simulink model "ans17"  (R2019a)
settings: Solver=VariableStepAuto  StartTime=0.0  StopTime=10.0  RelTol=1e-3
undefined symbols (not defined in the file or in its folder): a4, d1, feff, J_eff, KD, KI, KP, kT, n, TL
settings Model: Creator=andylei  LastModifiedBy=matth
settings DataIOCC: SaveFormat=StructureWithTime  ReturnWorkspaceOutputs=off
settings DebuggingCC: ArithmeticOperatorsInVariantConditions=warning

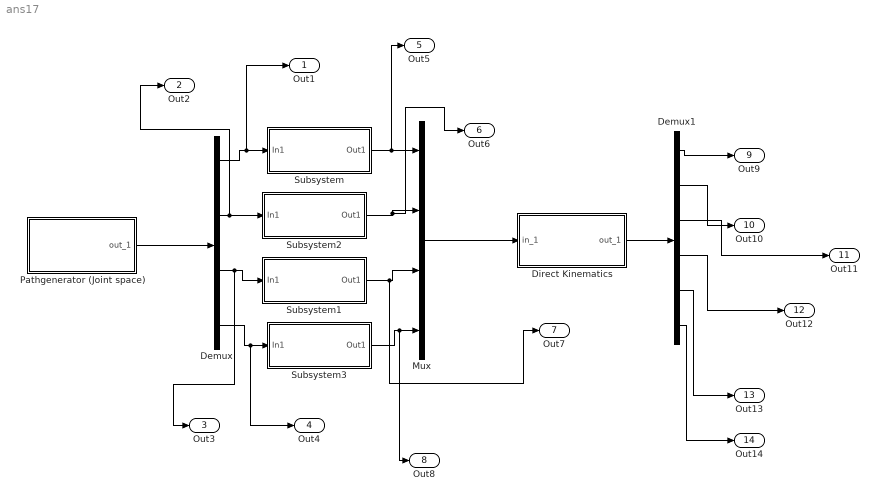
== system ans17 ==
  Demux : Demux
  Demux1 : Demux  Outputs=6
  Direct Kinematics : Subsystem
      mask Display: disp('Alto-Robot')
  Mux : Mux
  Pathgenerator (Joint space) : Subsystem
      mask Display: disp('Alto-Robot\n path -> q')
  Subsystem : Subsystem
  Subsystem1 : Subsystem
  Subsystem2 : Subsystem
  Subsystem3 : Subsystem
  Out1 : Outport
  Out2 : Outport  Port=2
  Out3 : Outport  Port=3
  Out4 : Outport  Port=4
  Out5 : Outport  Port=5
  Out6 : Outport  Port=6
  Out7 : Outport  Port=7
  Out8 : Outport  Port=8
  Out9 : Outport  Port=9
  Out10 : Outport  Port=10
  Out11 : Outport  Port=11
  Out12 : Outport  Port=12
  Out13 : Outport  Port=13
  Out14 : Outport  Port=14
  wires:
  Pathgenerator (Joint space)/1(out_1) -> Demux/1
  Mux/1 -> Direct Kinematics/1(in_1)
  Demux/1 -> Out1/1, Subsystem/1(In1)
  Demux/2 -> Subsystem2/1(In1), Out2/1
  Demux/3 -> Out3/1, Subsystem1/1(In1)
  Demux/4 -> Out4/1, Subsystem3/1(In1)
  Subsystem/1(Out1) -> Out5/1, Mux/1
  Subsystem2/1(Out1) -> Out6/1, Mux/2
  Subsystem1/1(Out1) -> Out7/1, Mux/3
  Subsystem3/1(Out1) -> Out8/1, Mux/4
  Direct Kinematics/1(out_1) -> Demux1/1
  Demux1/1 -> Out9/1
  Demux1/2 -> Out10/1
  Demux1/3 -> Out11/1
  Demux1/4 -> Out12/1
  Demux1/5 -> Out13/1
  Demux1/6 -> Out14/1

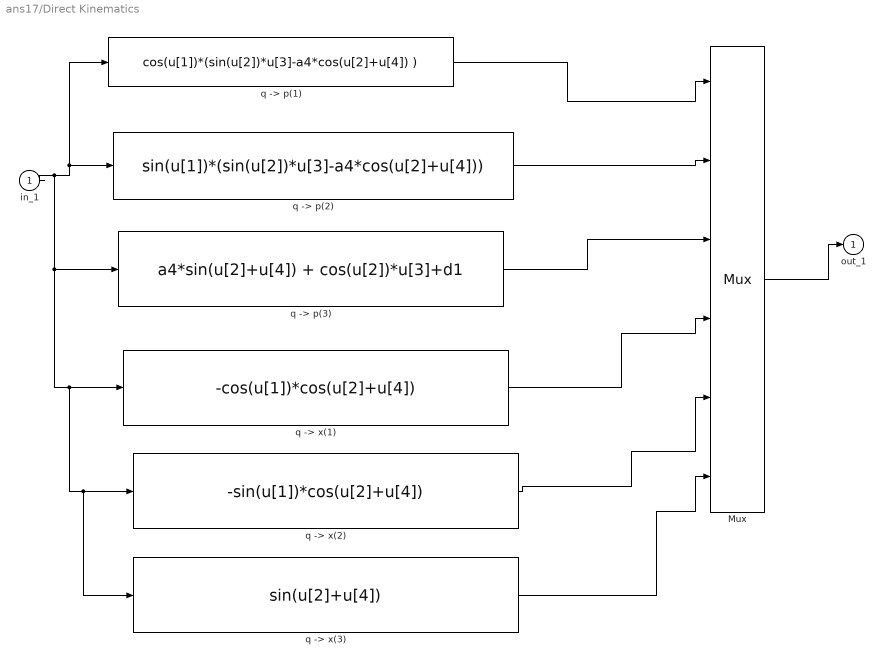
== system ans17/Direct Kinematics ==
  in_1 : Inport
  Mux : Mux  Inputs=6
  "q -> p(1)" : Fcn  Expr=cos(u[1])*(sin(u[2])*u[3]-a4*cos(u[2]+u[4]) )
  "q -> p(2)" : Fcn  Expr=sin(u[1])*(sin(u[2])*u[3]-a4*cos(u[2]+u[4]))
  "q -> p(3)" : Fcn  Expr=a4*sin(u[2]+u[4]) + cos(u[2])*u[3]+d1
  "q -> x(1)" : Fcn  Expr=-cos(u[1])*cos(u[2]+u[4])
  "q -> x(2)" : Fcn  Expr=-sin(u[1])*cos(u[2]+u[4])
  "q -> x(3)" : Fcn  Expr=sin(u[2]+u[4])
  out_1 : Outport  InitialOutput=0
  wires:
  Mux/1 -> out_1/1
  in_1/1 -> "q -> x(3)"/1, "q -> x(2)"/1, "q -> x(1)"/1, "q -> p(3)"/1, "q -> p(2)"/1, "q -> p(1)"/1
  "q -> x(3)"/1 -> Mux/6
  "q -> x(2)"/1 -> Mux/5
  "q -> x(1)"/1 -> Mux/4
  "q -> p(1)"/1 -> Mux/1
  "q -> p(2)"/1 -> Mux/2
  "q -> p(3)"/1 -> Mux/3

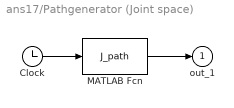
== system ans17/Pathgenerator (Joint space) ==
  Clock : Clock
  MATLAB Fcn : MATLABFcn  MATLABFcn=J_path  OutputDimensions=4
  out_1 : Outport
  wires:
  MATLAB Fcn/1 -> out_1/1
  Clock/1 -> MATLAB Fcn/1

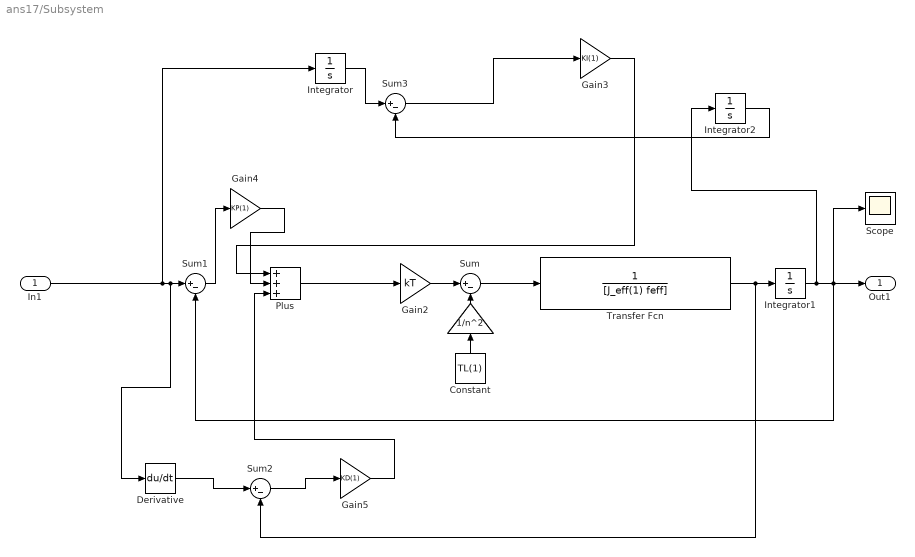
== system ans17/Subsystem ==
  In1 : Inport
  " " : Gain  Gain=1/n^2
  Constant : Constant  Value=TL(1)
  Derivative : Derivative
  Gain2 : Gain  Gain=kT
  Gain3 : Gain  Gain=KI(1)
  Gain4 : Gain  Gain=KP(1)
  Gain5 : Gain  Gain=KD(1)
  Integrator : Integrator
  Integrator1 : Integrator
  Integrator2 : Integrator
  Plus : Sum  Inputs=+++
  Scope : Scope
  Sum{,1..3} (4 alike) : Sum  Inputs=|+-
  Transfer Fcn : TransferFcn  Denominator=[J_eff(1) feff]
  Out1 : Outport
  wires:
  Sum3/1 -> Gain3/1
  Gain3/1 -> Plus/1
  Sum2/1 -> Gain5/1
  Integrator/1 -> Sum3/1
  Derivative/1 -> Sum2/1
  Gain5/1 -> Plus/3
  In1/1 -> Integrator/1, Derivative/1, Sum1/1
  Gain4/1 -> Plus/2
  Integrator1/1 -> Integrator2/1, Out1/1, Scope/1, Sum1/2
  Sum1/1 -> Gain4/1
  Gain2/1 -> Sum/1
  Transfer Fcn/1 -> Sum2/2, Integrator1/1
  Constant/1 -> " "/1
  " "/1 -> Sum/2
  Sum/1 -> Transfer Fcn/1
  Plus/1 -> Gain2/1
  Integrator2/1 -> Sum3/2

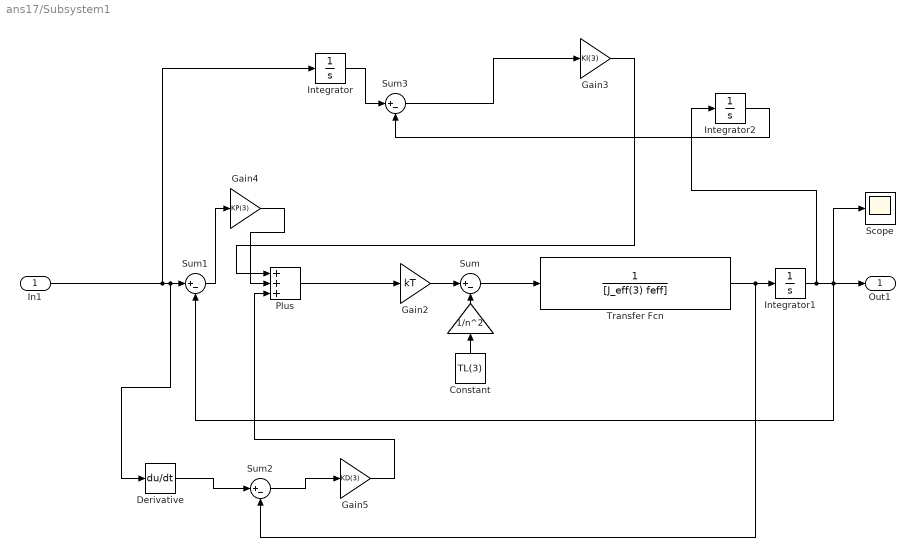
== system ans17/Subsystem1 ==
  In1 : Inport
  " " : Gain  Gain=1/n^2
  Constant : Constant  Value=TL(3)
  Derivative : Derivative
  Gain2 : Gain  Gain=kT
  Gain3 : Gain  Gain=KI(3)
  Gain4 : Gain  Gain=KP(3)
  Gain5 : Gain  Gain=KD(3)
  Integrator : Integrator
  Integrator1 : Integrator
  Integrator2 : Integrator
  Plus : Sum  Inputs=+++
  Scope : Scope
  Sum{,1..3} (4 alike) : Sum  Inputs=|+-
  Transfer Fcn : TransferFcn  Denominator=[J_eff(3) feff]
  Out1 : Outport
  wires:
  Sum3/1 -> Gain3/1
  Gain3/1 -> Plus/1
  Sum2/1 -> Gain5/1
  Integrator/1 -> Sum3/1
  Derivative/1 -> Sum2/1
  Gain5/1 -> Plus/3
  In1/1 -> Integrator/1, Derivative/1, Sum1/1
  Gain4/1 -> Plus/2
  Integrator1/1 -> Integrator2/1, Out1/1, Scope/1, Sum1/2
  Sum1/1 -> Gain4/1
  Gain2/1 -> Sum/1
  Transfer Fcn/1 -> Sum2/2, Integrator1/1
  Constant/1 -> " "/1
  " "/1 -> Sum/2
  Sum/1 -> Transfer Fcn/1
  Plus/1 -> Gain2/1
  Integrator2/1 -> Sum3/2

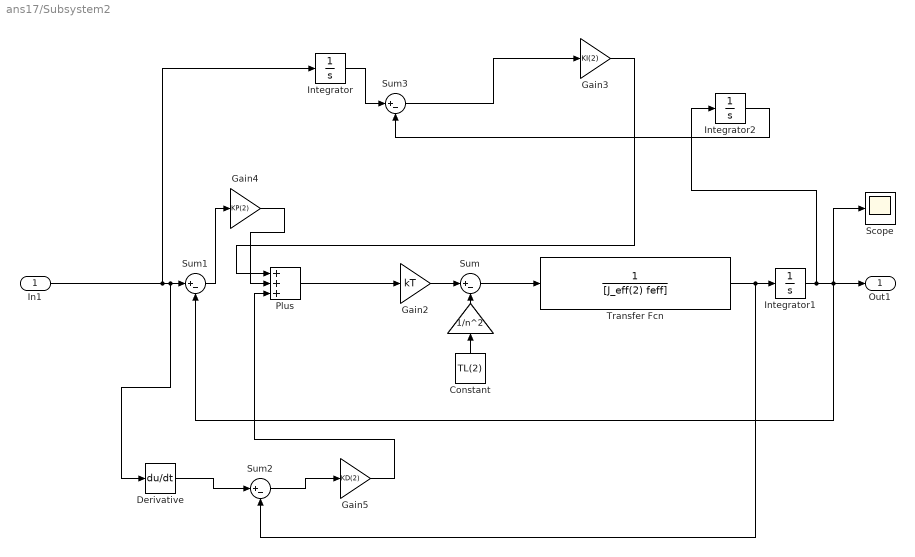
== system ans17/Subsystem2 ==
  In1 : Inport
  " " : Gain  Gain=1/n^2
  Constant : Constant  Value=TL(2)
  Derivative : Derivative
  Gain2 : Gain  Gain=kT
  Gain3 : Gain  Gain=KI(2)
  Gain4 : Gain  Gain=KP(2)
  Gain5 : Gain  Gain=KD(2)
  Integrator : Integrator
  Integrator1 : Integrator
  Integrator2 : Integrator
  Plus : Sum  Inputs=+++
  Scope : Scope
  Sum{,1..3} (4 alike) : Sum  Inputs=|+-
  Transfer Fcn : TransferFcn  Denominator=[J_eff(2) feff]
  Out1 : Outport
  wires:
  Sum3/1 -> Gain3/1
  Gain3/1 -> Plus/1
  Sum2/1 -> Gain5/1
  Integrator/1 -> Sum3/1
  Derivative/1 -> Sum2/1
  Gain5/1 -> Plus/3
  In1/1 -> Integrator/1, Derivative/1, Sum1/1
  Gain4/1 -> Plus/2
  Integrator1/1 -> Integrator2/1, Out1/1, Scope/1, Sum1/2
  Sum1/1 -> Gain4/1
  Gain2/1 -> Sum/1
  Transfer Fcn/1 -> Sum2/2, Integrator1/1
  Constant/1 -> " "/1
  " "/1 -> Sum/2
  Sum/1 -> Transfer Fcn/1
  Plus/1 -> Gain2/1
  Integrator2/1 -> Sum3/2

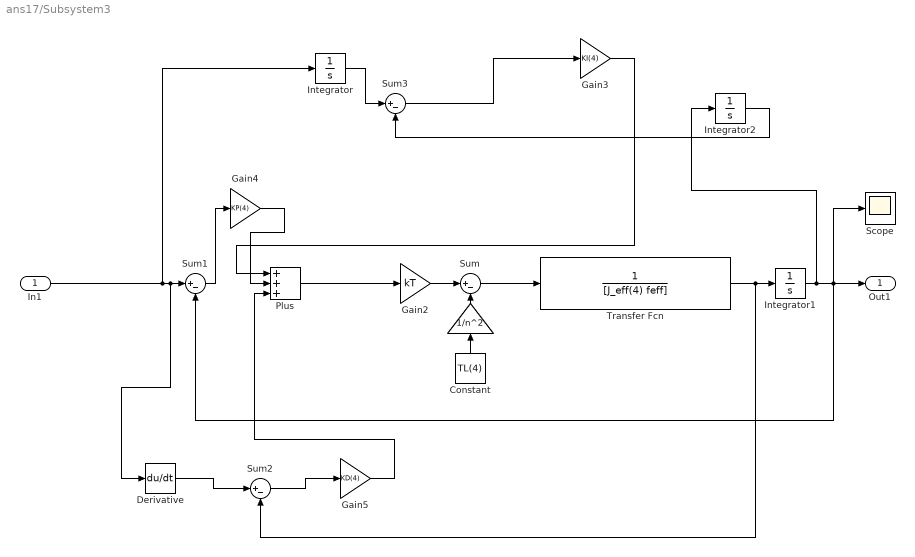
== system ans17/Subsystem3 ==
  In1 : Inport
  " " : Gain  Gain=1/n^2
  Constant : Constant  Value=TL(4)
  Derivative : Derivative
  Gain2 : Gain  Gain=kT
  Gain3 : Gain  Gain=KI(4)
  Gain4 : Gain  Gain=KP(4)
  Gain5 : Gain  Gain=KD(4)
  Integrator : Integrator
  Integrator1 : Integrator
  Integrator2 : Integrator
  Plus : Sum  Inputs=+++
  Scope : Scope
  Sum{,1..3} (4 alike) : Sum  Inputs=|+-
  Transfer Fcn : TransferFcn  Denominator=[J_eff(4) feff]
  Out1 : Outport
  wires:
  Sum3/1 -> Gain3/1
  Gain3/1 -> Plus/1
  Sum2/1 -> Gain5/1
  Integrator/1 -> Sum3/1
  Derivative/1 -> Sum2/1
  Gain5/1 -> Plus/3
  In1/1 -> Integrator/1, Derivative/1, Sum1/1
  Gain4/1 -> Plus/2
  Integrator1/1 -> Integrator2/1, Out1/1, Scope/1, Sum1/2
  Sum1/1 -> Gain4/1
  Gain2/1 -> Sum/1
  Transfer Fcn/1 -> Sum2/2, Integrator1/1
  Constant/1 -> " "/1
  " "/1 -> Sum/2
  Sum/1 -> Transfer Fcn/1
  Plus/1 -> Gain2/1
  Integrator2/1 -> Sum3/2
